simulink model "EvPowertrainController2EM"  (R2022b)
settings: configuration reference "VehicleFixed10ms" (kept outside this file)
model workspace (MAT data in the model file):
  CtrlVcuCnstrntPnltyFctr = 10000000
  CtrlVcuEMTrqSplitGrid = 200
  CtrlVcuPwrDeltaPnlty = 2
  CtrlVcuTracPwrErrPnlty = 6
  CtrlVcuTrqVecBrkThresh = 0.01
  CtrlVcuTrqVecIGain = 0
  CtrlVcuTrqVecMinTrq = 50
  CtrlVcuTrqVecPGain = -2000
  CtrlVcuTrqVecSteerThresh = 0.349065850399
  CtrlVcuTrqVecVelThresh = 2.5
undefined symbols (not defined in the file): AAM_IM_InvGrbx_Ploss, AAM_IM_spd, AAM_IM_TrqBrkPts, AAM_IPM_InvGrbx_Ploss, AAM_IPM_spd, AAM_IPM_TrqBrkPts, Bolt_n_map_spd, Bolt_n_map_trq, BrkPts_Spd, BrkPts_Trq, BrkPts_Vdc, CtrlVcuEvChrgLmtBpt, CtrlVcuEvRegenBrkCutOff, CtrlVcuEvRegenBrkSpdBpt, CtrlVcuEvSocBpt, eff, FrontDiffRatio, PlntBrkActrBoreFrnt, PlntBrkFrntBias, PlntBrkKinFricCffFrnt, PlntBrkNumPadsFrnt, PlntBrkPadMeanRadiusFrnt, PlntBrkPrsFctr, PlntBrkRearBias, PlntDiffrntl2Eff, PlntDiffrntl2Ratio, PlntDiffrntlEff, PlntDiffrntlRatio, PlntEM3Trq, PlntEMWhlGearEffFL, PlntEMWhlGearEffRL, PlntEMWhlGearRatioFL, PlntEMWhlGearRatioRL, PlntTransEffSpdBpt, PlntTransEffTbl, PlntTransEffTempBpt, PlntTransEffTrqBpt, PlntTransGearNumVect, PlntTransGearRatioVect, PlntWhlLdRadius, Ploss_AllVdc, RearDiffRatio, Spark_EffMap, Spark_MaxTrq, Spark_MaxTrq_Spd, Spark_Spd_BrkPts, Spark_Trq_BrkPts, SRM_DCVoltBrkPnt, SRM_InvGrbx_Ploss, SRM_op_TrqBrkPnt, SRM_Ploss_InvMotGrbx, SRM_SpdBrkPnt, SRM_TrqBrkPnt
libraries: simulink x7, autolibutils x2
(part 2 of 2)

== system EvPowertrainController2EM/Energy Management/Convert Whl to EMTrq Vector/2EM/Diff Eta1 ==
  note: Pwr >= 0, v = 1
      | Pwr < 0, v= -1
  SpdIn : Inport
  TrqIn : Inport  Port=2
  Constant : Constant  Value=PlntDiffrntl2Eff
  Constant1 : Constant  SampleTime=-1
  Constant2 : Constant  Value=-1  SampleTime=-1
  Math Function1 : Math  Operator=pow  SignedPower=on  OutputSignalType=real
  Product1 : Product
  Switch2 : Switch  SaturateOnIntegerOverflow=off  InputSameDT=off
  eta : Outport  VectorParamsAs1DForOutWhenUnconnected=off
  wires:
  TrqIn/1 -> Product1/1
  Math Function1/1 -> eta/1
  Switch2/1 -> Math Function1/2
  Product1/1 -> Switch2/2
  Constant1/1 -> Switch2/1
  Constant2/1 -> Switch2/3
  Constant/1 -> Math Function1/1
  SpdIn/1 -> Product1/2

== system EvPowertrainController2EM/Energy Management/Convert Whl to EMTrq Vector/3EM Dual Front/Diff Eta ==
  note: Pwr >= 0, v = 1
      | Pwr < 0, v= -1
  SpdIn : Inport
  TrqIn : Inport  Port=2
  Constant : Constant  Value=PlntDiffrntl2Eff
  Constant1 : Constant  SampleTime=-1
  Constant2 : Constant  Value=-1  SampleTime=-1
  Math Function1 : Math  Operator=pow  SignedPower=on  OutputSignalType=real
  Product1 : Product
  Switch2 : Switch  SaturateOnIntegerOverflow=off  InputSameDT=off
  eta : Outport  VectorParamsAs1DForOutWhenUnconnected=off
  wires:
  SpdIn/1 -> Product1/2
  Constant/1 -> Math Function1/1
  Constant2/1 -> Switch2/3
  Constant1/1 -> Switch2/1
  Product1/1 -> Switch2/2
  Switch2/1 -> Math Function1/2
  Math Function1/1 -> eta/1
  TrqIn/1 -> Product1/1

== system EvPowertrainController2EM/Energy Management/Convert Whl to EMTrq Vector/3EM Dual Front/Gear Eta ==
  note: Pwr >= 0, v = 1
      | Pwr < 0, v= -1
  SpdIn : Inport
  TrqIn : Inport  Port=2
  Constant : Constant  Value=PlntEMWhlGearEffFL
  Constant1 : Constant  SampleTime=-1
  Constant2 : Constant  Value=-1  SampleTime=-1
  Math Function1 : Math  Operator=pow  SignedPower=on  OutputSignalType=real
  Product1 : Product
  Switch2 : Switch  SaturateOnIntegerOverflow=off  InputSameDT=off
  eta : Outport  VectorParamsAs1DForOutWhenUnconnected=off
  wires:
  TrqIn/1 -> Product1/1
  Math Function1/1 -> eta/1
  Switch2/1 -> Math Function1/2
  Product1/1 -> Switch2/2
  Constant1/1 -> Switch2/1
  Constant2/1 -> Switch2/3
  Constant/1 -> Math Function1/1
  SpdIn/1 -> Product1/2

== system EvPowertrainController2EM/Energy Management/Convert Whl to EMTrq Vector/3EM Dual Rear/Diff Eta ==
  note: Pwr >= 0, v = 1
      | Pwr < 0, v= -1
  SpdIn : Inport
  TrqIn : Inport  Port=2
  Constant : Constant  Value=PlntDiffrntlEff
  Constant1 : Constant  SampleTime=-1
  Constant2 : Constant  Value=-1  SampleTime=-1
  Math Function1 : Math  Operator=pow  SignedPower=on  OutputSignalType=real
  Product1 : Product
  Switch2 : Switch  SaturateOnIntegerOverflow=off  InputSameDT=off
  eta : Outport  VectorParamsAs1DForOutWhenUnconnected=off
  wires:
  SpdIn/1 -> Product1/2
  Constant/1 -> Math Function1/1
  Constant2/1 -> Switch2/3
  Constant1/1 -> Switch2/1
  Product1/1 -> Switch2/2
  Switch2/1 -> Math Function1/2
  Math Function1/1 -> eta/1
  TrqIn/1 -> Product1/1

== system EvPowertrainController2EM/Energy Management/Convert Whl to EMTrq Vector/3EM Dual Rear/Gear Eta ==
  note: Pwr >= 0, v = 1
      | Pwr < 0, v= -1
  SpdIn : Inport
  TrqIn : Inport  Port=2
  Constant : Constant  Value=PlntEMWhlGearEffRL
  Constant1 : Constant  SampleTime=-1
  Constant2 : Constant  Value=-1  SampleTime=-1
  Math Function1 : Math  Operator=pow  SignedPower=on  OutputSignalType=real
  Product1 : Product
  Switch2 : Switch  SaturateOnIntegerOverflow=off  InputSameDT=off
  eta : Outport  VectorParamsAs1DForOutWhenUnconnected=off
  wires:
  TrqIn/1 -> Product1/1
  Math Function1/1 -> eta/1
  Switch2/1 -> Math Function1/2
  Product1/1 -> Switch2/2
  Constant1/1 -> Switch2/1
  Constant2/1 -> Switch2/3
  Constant/1 -> Math Function1/1
  SpdIn/1 -> Product1/2

== system EvPowertrainController2EM/Energy Management/Convert Whl to EMTrq Vector/4EM/Gear Eta ==
  note: Pwr >= 0, v = 1
      | Pwr < 0, v= -1
  SpdIn : Inport
  TrqIn : Inport  Port=2
  Constant : Constant  Value=PlntEMWhlGearEffFL
  Constant1 : Constant  SampleTime=-1
  Constant2 : Constant  Value=-1  SampleTime=-1
  Math Function1 : Math  Operator=pow  SignedPower=on  OutputSignalType=real
  Product1 : Product
  Switch2 : Switch  SaturateOnIntegerOverflow=off  InputSameDT=off
  eta : Outport  VectorParamsAs1DForOutWhenUnconnected=off
  wires:
  TrqIn/1 -> Product1/1
  Math Function1/1 -> eta/1
  Switch2/1 -> Math Function1/2
  Product1/1 -> Switch2/2
  Constant1/1 -> Switch2/1
  Constant2/1 -> Switch2/3
  Constant/1 -> Math Function1/1
  SpdIn/1 -> Product1/2

== system EvPowertrainController2EM/Energy Management/Convert Whl to EMTrq Vector/4EM/Gear Eta1 ==
  note: Pwr >= 0, v = 1
      | Pwr < 0, v= -1
  SpdIn : Inport
  TrqIn : Inport  Port=2
  Constant : Constant  Value=PlntEMWhlGearEffRL
  Constant1 : Constant  SampleTime=-1
  Constant2 : Constant  Value=-1  SampleTime=-1
  Math Function1 : Math  Operator=pow  SignedPower=on  OutputSignalType=real
  Product1 : Product
  Switch2 : Switch  SaturateOnIntegerOverflow=off  InputSameDT=off
  eta : Outport  VectorParamsAs1DForOutWhenUnconnected=off
  wires:
  SpdIn/1 -> Product1/2
  Constant/1 -> Math Function1/1
  Constant2/1 -> Switch2/3
  Constant1/1 -> Switch2/1
  Product1/1 -> Switch2/2
  Switch2/1 -> Math Function1/2
  Math Function1/1 -> eta/1
  TrqIn/1 -> Product1/1

== system EvPowertrainController2EM/Energy Management/Powertrain Constraints /Battery Constraint/Electrical Current ==
  BattV : Inport
  EMPwrElecVec : Inport  Port=2
  DC-DC Eta : Subsystem  Variant=on  VariantControlMode=label  VariantControl=Variant1  LabelModeActiveChoice=0
  Divide : Product  Inputs=*/
  Saturation : Saturate  UpperLimit=Inf  LowerLimit=0.0001
  BatteryAmp : Outport  VectorParamsAs1DForOutWhenUnconnected=off
  wires:
  DC-DC Eta/1(Out) -> Divide/1
  EMPwrElecVec/1 -> DC-DC Eta/1(In)
  Divide/1 -> BatteryAmp/1
  BattV/1 -> Saturation/1
  Saturation/1 -> Divide/2

== system EvPowertrainController2EM/Energy Management/Powertrain Constraints /Battery Constraint/Power Limit Calculations ==
  note: Use Current Limits from BMS to calculate
      | discharge and charge power limits
  BattPwrDisChrgLmt : Inport
  "BattPwrChrgLmt " : Inport  Port=2
  BattV_in : Inport  Port=3
  Data Type Conversion : DataTypeConversion  SaturateOnIntegerOverflow=off  RndMeth=Floor
  Data Type Conversion1 : DataTypeConversion  SaturateOnIntegerOverflow=off  RndMeth=Floor
  Divide : Product  Inputs=*/
  Divide1 : Product  Inputs=/*
  div0protect - poly : autolibutils/div0protect - poly  thresh=.01  ZeroCross=off  ZeroCross1=on  aMode=aMode
  div0protect - poly1 : autolibutils/div0protect - poly  thresh=.01  ZeroCross=off  ZeroCross1=on  aMode=aMode
  BattCurrDischrgLmt : Outport  VectorParamsAs1DForOutWhenUnconnected=off
  BattCurrChrgLmt : Outport  Port=2  VectorParamsAs1DForOutWhenUnconnected=off
  BattPwrDischrgLmt : Outport  Port=3  VectorParamsAs1DForOutWhenUnconnected=off
  BattPwrChrgLmt : Outport  Port=4  VectorParamsAs1DForOutWhenUnconnected=off
  wires:
  "BattPwrChrgLmt "/1 -> Divide1/2, Data Type Conversion/1
  BattPwrDisChrgLmt/1 -> Divide/1, Data Type Conversion1/1
  Data Type Conversion/1 -> BattPwrChrgLmt/1
  Data Type Conversion1/1 -> BattPwrDischrgLmt/1
  Divide/1 -> BattCurrDischrgLmt/1
  BattV_in/1 -> div0protect - poly/1, div0protect - poly1/1
  Divide1/1 -> BattCurrChrgLmt/1
  div0protect - poly/1 -> Divide1/1
  div0protect - poly1/1 -> Divide/2

== system EvPowertrainController2EM/Energy Management/Powertrain Constraints /EM Constraint Front/Maximum Torque ==
  note: Don't allow negative MotTrq when
      | WhlTrqCmd is >= 0
  WhlTrqCmd : Inport
  WhlEMTrqSplitVecFrnt : Inport  Port=2
  WhlTrqMaxVec : Inport  Port=3
  Compare To Zero : simulink/Logic and Bit Operations/Compare To Zero  relop=<  OutDataTypeStr=boolean
  Compare To Zero1 : simulink/Logic and Bit Operations/Compare To Zero  relop=>=  OutDataTypeStr=boolean
  Gain : Gain  Gain=-1
  Logical Operator : Logic  Operator=OR  Inputs=3  AllPortsSameDT=off  OutDataTypeStr=boolean
  Logical Operator1 : Logic  AllPortsSameDT=off  OutDataTypeStr=boolean
  Relational Operator : RelationalOperator  Operator=<  OutDataTypeStr=boolean  RndMeth=Simplest  InputSameDT=off
  Relational Operator1 : RelationalOperator  Operator=<  OutDataTypeStr=boolean  RndMeth=Simplest  InputSameDT=off
  Saturation Dynamic : simulink/Discontinuities/Saturation Dynamic  OutMin=[]  OutMax=[]  OutDataTypeStr=Inherit: Same as second input  OutDataType=fixdt(1, 16)  OutScaling=2^-10  DoSatur=off
  WhlEMTrqSatVec : Outport  VectorParamsAs1DForOutWhenUnconnected=off
  InfeasibleEMVec : Outport  Port=2  VectorParamsAs1DForOutWhenUnconnected=off
  wires:
  Logical Operator1/1 -> Logical Operator/3
  Compare To Zero1/1 -> Logical Operator1/2
  WhlEMTrqSplitVecFrnt/1 -> Relational Operator/2, Relational Operator1/1, Saturation Dynamic/2, Compare To Zero/1
  Compare To Zero/1 -> Logical Operator1/1
  WhlTrqCmd/1 -> Compare To Zero1/1
  Gain/1 -> Relational Operator1/2, Saturation Dynamic/3
  Saturation Dynamic/1 -> WhlEMTrqSatVec/1
  Relational Operator/1 -> Logical Operator/1
  Relational Operator1/1 -> Logical Operator/2
  Logical Operator/1 -> InfeasibleEMVec/1
  WhlTrqMaxVec/1 -> Gain/1, Relational Operator/1, Saturation Dynamic/1

== system EvPowertrainController2EM/Energy Management/Powertrain Constraints /EM Constraint Front/Tabular Power Loss Data ==
  EMAvgSpdVec : Inport
  WhlEMTrqSatVec : Inport  Port=2
  BatVin : Inport  Port=3
  2EM Stock : Subsystem  VariantControl=FrEff == 1
  2EM Team : Subsystem  VariantControl=FrEff == 2
  EMPwrElecVec : Outport

== system EvPowertrainController2EM/Energy Management/Powertrain Constraints /EM Constraint Rear/Maximum Torque ==
  note: Don't allow negative MotTrq when
      | WhlTrqCmd is >= 0
  WhlTrqCmd : Inport
  WhlEMTrqSplitVecRear : Inport  Port=2
  WhlTrqMaxVec : Inport  Port=3
  Compare To Zero : simulink/Logic and Bit Operations/Compare To Zero  relop=<  OutDataTypeStr=boolean
  Compare To Zero1 : simulink/Logic and Bit Operations/Compare To Zero  relop=>=  OutDataTypeStr=boolean
  Gain : Gain  Gain=-1
  Logical Operator : Logic  Operator=OR  Inputs=3  AllPortsSameDT=off  OutDataTypeStr=boolean
  Logical Operator1 : Logic  AllPortsSameDT=off  OutDataTypeStr=boolean
  Relational Operator : RelationalOperator  Operator=<  OutDataTypeStr=boolean  RndMeth=Simplest  InputSameDT=off
  Relational Operator1 : RelationalOperator  Operator=<  OutDataTypeStr=boolean  RndMeth=Simplest  InputSameDT=off
  Saturation Dynamic : simulink/Discontinuities/Saturation Dynamic  OutMin=[]  OutMax=[]  OutDataTypeStr=Inherit: Same as second input  OutDataType=fixdt(1, 16)  OutScaling=2^-10  DoSatur=off
  WhlEMTrqSatVec : Outport  VectorParamsAs1DForOutWhenUnconnected=off
  InfeasibleEMVec : Outport  Port=2  VectorParamsAs1DForOutWhenUnconnected=off
  wires:
  WhlTrqMaxVec/1 -> Saturation Dynamic/1, Relational Operator/1, Gain/1
  Logical Operator/1 -> InfeasibleEMVec/1
  Relational Operator1/1 -> Logical Operator/2
  Relational Operator/1 -> Logical Operator/1
  Saturation Dynamic/1 -> WhlEMTrqSatVec/1
  Gain/1 -> Saturation Dynamic/3, Relational Operator1/2
  WhlTrqCmd/1 -> Compare To Zero1/1
  Compare To Zero/1 -> Logical Operator1/1
  WhlEMTrqSplitVecRear/1 -> Compare To Zero/1, Saturation Dynamic/2, Relational Operator1/1, Relational Operator/2
  Compare To Zero1/1 -> Logical Operator1/2
  Logical Operator1/1 -> Logical Operator/3

== system EvPowertrainController2EM/Energy Management/Powertrain Constraints /EM Constraint Rear/Tabular Power Loss Data ==
  EMAvgSpdVec : Inport
  WhlEMTrqSatVec : Inport  Port=2
  BatVin : Inport  Port=3
  2EM Stock : Subsystem  VariantControl=RrEff == 1
  2EM Team : Subsystem  VariantControl=RrEff == 2
  EMPwrElecVec : Outport

== system EvPowertrainController2EM/Accel Pedal to Traction Wheel Torque Request/2EM/EMTrq2WhlTrqFrnt/No Transmission/Diff Eta ==
  note: Pwr >= 0, v = 1
      | Pwr < 0, v= -1
  SpdIn : Inport
  TrqIn : Inport  Port=2
  Constant : Constant  Value=PlntDiffrntlEff
  Constant1 : Constant  SampleTime=-1
  Constant2 : Constant  Value=-1  SampleTime=-1
  Math Function1 : Math  Operator=pow  SignedPower=on  OutputSignalType=real
  Product1 : Product
  Switch2 : Switch  SaturateOnIntegerOverflow=off  InputSameDT=off
  eta : Outport  VectorParamsAs1DForOutWhenUnconnected=off
  wires:
  SpdIn/1 -> Product1/2
  Constant/1 -> Math Function1/1
  Constant2/1 -> Switch2/3
  Constant1/1 -> Switch2/1
  Product1/1 -> Switch2/2
  Switch2/1 -> Math Function1/2
  Math Function1/1 -> eta/1
  TrqIn/1 -> Product1/1

== system EvPowertrainController2EM/Accel Pedal to Traction Wheel Torque Request/2EM/EMTrq2WhlTrqFrnt/Transmission/Diff Eta ==
  SpdIn : Inport
  TrqIn : Inport  Port=2
  Constant : Constant  Value=PlntDiffrntlEff
  Constant1 : Constant  SampleTime=-1
  Constant2 : Constant  Value=-1  SampleTime=-1
  Math Function1 : Math  Operator=pow  SignedPower=on  OutputSignalType=real
  Product1 : Product
  Switch2 : Switch  SaturateOnIntegerOverflow=off  InputSameDT=off
  eta : Outport  VectorParamsAs1DForOutWhenUnconnected=off
  wires:
  SpdIn/1 -> Product1/2
  Constant/1 -> Math Function1/1
  Constant2/1 -> Switch2/3
  Constant1/1 -> Switch2/1
  Product1/1 -> Switch2/2
  Switch2/1 -> Math Function1/2
  Math Function1/1 -> eta/1
  TrqIn/1 -> Product1/1

== system EvPowertrainController2EM/Accel Pedal to Traction Wheel Torque Request/2EM/EMTrq2WhlTrqFrnt/Transmission/Trans Eta ==
  TrqIn : Inport
  SpdIn : Inport  Port=2
  Gear : Inport  Port=3
  Abs1 : Abs  SaturateOnIntegerOverflow=off
  Constant : Constant  Value=PlntTransEffTempBpt(1)
  Constant1 : Constant  SampleTime=-1
  Constant2 : Constant  Value=-1  SampleTime=-1
  Eta 4D : Lookup_n-D  NumberOfTableDimensions=4  LookupTableObject=''  BreakpointsForDimension1=PlntTransEffTrqBpt  BreakpointsForDimension2=PlntTransEffSpdBpt  BreakpointsForDimension3=PlntTransGearNumVect  BreakpointsForDimension4=PlntTransEffTempBpt  Table=PlntTransEffTbl  ExtrapMethod=Clip  InternalRulePriority=Speed  RndMeth=Simplest
      settings: InputPortMap=u0,u1,u2,u3
  Math Function1 : Math  Operator=pow  SignedPower=on  OutputSignalType=real
  Product1 : Product
  Switch2 : Switch  SaturateOnIntegerOverflow=off  InputSameDT=off
  eta : Outport  VectorParamsAs1DForOutWhenUnconnected=off
  wires:
  TrqIn/1 -> Product1/1, Abs1/1
  Math Function1/1 -> eta/1
  Abs1/1 -> Eta 4D/1
  Switch2/1 -> Math Function1/2
  Product1/1 -> Switch2/2
  Constant1/1 -> Switch2/1
  Constant2/1 -> Switch2/3
  Eta 4D/1 -> Math Function1/1
  SpdIn/1 -> Product1/2, Eta 4D/2
  Gear/1 -> Eta 4D/3
  Constant/1 -> Eta 4D/4

== system EvPowertrainController2EM/Accel Pedal to Traction Wheel Torque Request/2EM/EMTrq2WhlTrqRear/No Transmission/Diff Eta ==
  note: Pwr >= 0, v = 1
      | Pwr < 0, v= -1
  SpdIn : Inport
  TrqIn : Inport  Port=2
  Constant : Constant  Value=PlntDiffrntl2Eff
  Constant1 : Constant  SampleTime=-1
  Constant2 : Constant  Value=-1  SampleTime=-1
  Math Function1 : Math  Operator=pow  SignedPower=on  OutputSignalType=real
  Product1 : Product
  Switch2 : Switch  SaturateOnIntegerOverflow=off  InputSameDT=off
  eta : Outport  VectorParamsAs1DForOutWhenUnconnected=off
  wires:
  SpdIn/1 -> Product1/2
  Constant/1 -> Math Function1/1
  Constant2/1 -> Switch2/3
  Constant1/1 -> Switch2/1
  Product1/1 -> Switch2/2
  Switch2/1 -> Math Function1/2
  Math Function1/1 -> eta/1
  TrqIn/1 -> Product1/1

== system EvPowertrainController2EM/Accel Pedal to Traction Wheel Torque Request/2EM/EMTrq2WhlTrqRear/Transmission/Diff Eta ==
  SpdIn : Inport
  TrqIn : Inport  Port=2
  Constant : Constant  Value=PlntDiffrntl2Eff
  Constant1 : Constant  SampleTime=-1
  Constant2 : Constant  Value=-1  SampleTime=-1
  Math Function1 : Math  Operator=pow  SignedPower=on  OutputSignalType=real
  Product1 : Product
  Switch2 : Switch  SaturateOnIntegerOverflow=off  InputSameDT=off
  eta : Outport  VectorParamsAs1DForOutWhenUnconnected=off
  wires:
  TrqIn/1 -> Product1/1
  Math Function1/1 -> eta/1
  Switch2/1 -> Math Function1/2
  Product1/1 -> Switch2/2
  Constant1/1 -> Switch2/1
  Constant2/1 -> Switch2/3
  Constant/1 -> Math Function1/1
  SpdIn/1 -> Product1/2

== system EvPowertrainController2EM/Accel Pedal to Traction Wheel Torque Request/2EM/EMTrq2WhlTrqRear/Transmission/Trans Eta ==
  TrqIn : Inport
  SpdIn : Inport  Port=2
  Gear : Inport  Port=3
  Abs1 : Abs  SaturateOnIntegerOverflow=off
  Constant : Constant  Value=PlntTransEffTempBpt(1)
  Constant1 : Constant  SampleTime=-1
  Constant2 : Constant  Value=-1  SampleTime=-1
  Eta 4D : Lookup_n-D  NumberOfTableDimensions=4  LookupTableObject=''  BreakpointsForDimension1=PlntTransEffTrqBpt  BreakpointsForDimension2=PlntTransEffSpdBpt  BreakpointsForDimension3=PlntTransGearNumVect  BreakpointsForDimension4=PlntTransEffTempBpt  Table=PlntTransEffTbl  ExtrapMethod=Clip  InternalRulePriority=Speed  RndMeth=Simplest
      settings: InputPortMap=u0,u1,u2,u3
  Math Function1 : Math  Operator=pow  SignedPower=on  OutputSignalType=real
  Product1 : Product
  Switch2 : Switch  SaturateOnIntegerOverflow=off  InputSameDT=off
  eta : Outport  VectorParamsAs1DForOutWhenUnconnected=off
  wires:
  Constant/1 -> Eta 4D/4
  Gear/1 -> Eta 4D/3
  SpdIn/1 -> Eta 4D/2, Product1/2
  Eta 4D/1 -> Math Function1/1
  Constant2/1 -> Switch2/3
  Constant1/1 -> Switch2/1
  Product1/1 -> Switch2/2
  Switch2/1 -> Math Function1/2
  Abs1/1 -> Eta 4D/1
  Math Function1/1 -> eta/1
  TrqIn/1 -> Abs1/1, Product1/1

== system EvPowertrainController2EM/Energy Management/2EM/EMTrq2WhlTrqFrnt/No Transmission/Diff Eta ==
  note: Pwr >= 0, v = 1
      | Pwr < 0, v= -1
  SpdIn : Inport
  TrqIn : Inport  Port=2
  Constant : Constant  Value=PlntDiffrntlEff
  Constant1 : Constant  SampleTime=-1
  Constant2 : Constant  Value=-1  SampleTime=-1
  Math Function1 : Math  Operator=pow  SignedPower=on  OutputSignalType=real
  Product1 : Product
  Switch2 : Switch  SaturateOnIntegerOverflow=off  InputSameDT=off
  eta : Outport  VectorParamsAs1DForOutWhenUnconnected=off
  wires:
  SpdIn/1 -> Product1/2
  Constant/1 -> Math Function1/1
  Constant2/1 -> Switch2/3
  Constant1/1 -> Switch2/1
  Product1/1 -> Switch2/2
  Switch2/1 -> Math Function1/2
  Math Function1/1 -> eta/1
  TrqIn/1 -> Product1/1

== system EvPowertrainController2EM/Energy Management/2EM/EMTrq2WhlTrqFrnt/Transmission/Diff Eta ==
  SpdIn : Inport
  TrqIn : Inport  Port=2
  Constant : Constant  Value=PlntDiffrntlEff
  Constant1 : Constant  SampleTime=-1
  Constant2 : Constant  Value=-1  SampleTime=-1
  Math Function1 : Math  Operator=pow  SignedPower=on  OutputSignalType=real
  Product1 : Product
  Switch2 : Switch  SaturateOnIntegerOverflow=off  InputSameDT=off
  eta : Outport  VectorParamsAs1DForOutWhenUnconnected=off
  wires:
  SpdIn/1 -> Product1/2
  Constant/1 -> Math Function1/1
  Constant2/1 -> Switch2/3
  Constant1/1 -> Switch2/1
  Product1/1 -> Switch2/2
  Switch2/1 -> Math Function1/2
  Math Function1/1 -> eta/1
  TrqIn/1 -> Product1/1

== system EvPowertrainController2EM/Energy Management/2EM/EMTrq2WhlTrqFrnt/Transmission/Trans Eta ==
  TrqIn : Inport
  SpdIn : Inport  Port=2
  Gear : Inport  Port=3
  Abs1 : Abs  SaturateOnIntegerOverflow=off
  Constant : Constant  Value=PlntTransEffTempBpt(1)
  Constant1 : Constant  SampleTime=-1
  Constant2 : Constant  Value=-1  SampleTime=-1
  Eta 4D : Lookup_n-D  NumberOfTableDimensions=4  LookupTableObject=''  BreakpointsForDimension1=PlntTransEffTrqBpt  BreakpointsForDimension2=PlntTransEffSpdBpt  BreakpointsForDimension3=PlntTransGearNumVect  BreakpointsForDimension4=PlntTransEffTempBpt  Table=PlntTransEffTbl  ExtrapMethod=Clip  InternalRulePriority=Speed  RndMeth=Simplest
      settings: InputPortMap=u0,u1,u2,u3
  Math Function1 : Math  Operator=pow  SignedPower=on  OutputSignalType=real
  Product1 : Product
  Switch2 : Switch  SaturateOnIntegerOverflow=off  InputSameDT=off
  eta : Outport  VectorParamsAs1DForOutWhenUnconnected=off
  wires:
  TrqIn/1 -> Product1/1, Abs1/1
  Math Function1/1 -> eta/1
  Abs1/1 -> Eta 4D/1
  Switch2/1 -> Math Function1/2
  Product1/1 -> Switch2/2
  Constant1/1 -> Switch2/1
  Constant2/1 -> Switch2/3
  Eta 4D/1 -> Math Function1/1
  SpdIn/1 -> Product1/2, Eta 4D/2
  Gear/1 -> Eta 4D/3
  Constant/1 -> Eta 4D/4

== system EvPowertrainController2EM/Energy Management/2EM/EMTrq2WhlTrqRear/No Transmission/Diff Eta ==
  note: Pwr >= 0, v = 1
      | Pwr < 0, v= -1
  SpdIn : Inport
  TrqIn : Inport  Port=2
  Constant : Constant  Value=PlntDiffrntl2Eff
  Constant1 : Constant  SampleTime=-1
  Constant2 : Constant  Value=-1  SampleTime=-1
  Math Function1 : Math  Operator=pow  SignedPower=on  OutputSignalType=real
  Product1 : Product
  Switch2 : Switch  SaturateOnIntegerOverflow=off  InputSameDT=off
  eta : Outport  VectorParamsAs1DForOutWhenUnconnected=off
  wires:
  SpdIn/1 -> Product1/2
  Constant/1 -> Math Function1/1
  Constant2/1 -> Switch2/3
  Constant1/1 -> Switch2/1
  Product1/1 -> Switch2/2
  Switch2/1 -> Math Function1/2
  Math Function1/1 -> eta/1
  TrqIn/1 -> Product1/1

== system EvPowertrainController2EM/Energy Management/2EM/EMTrq2WhlTrqRear/Transmission/Diff Eta ==
  SpdIn : Inport
  TrqIn : Inport  Port=2
  Constant : Constant  Value=PlntDiffrntl2Eff
  Constant1 : Constant  SampleTime=-1
  Constant2 : Constant  Value=-1  SampleTime=-1
  Math Function1 : Math  Operator=pow  SignedPower=on  OutputSignalType=real
  Product1 : Product
  Switch2 : Switch  SaturateOnIntegerOverflow=off  InputSameDT=off
  eta : Outport  VectorParamsAs1DForOutWhenUnconnected=off
  wires:
  TrqIn/1 -> Product1/1
  Math Function1/1 -> eta/1
  Switch2/1 -> Math Function1/2
  Product1/1 -> Switch2/2
  Constant1/1 -> Switch2/1
  Constant2/1 -> Switch2/3
  Constant/1 -> Math Function1/1
  SpdIn/1 -> Product1/2

== system EvPowertrainController2EM/Energy Management/2EM/EMTrq2WhlTrqRear/Transmission/Trans Eta ==
  TrqIn : Inport
  SpdIn : Inport  Port=2
  Gear : Inport  Port=3
  Abs1 : Abs  SaturateOnIntegerOverflow=off
  Constant : Constant  Value=PlntTransEffTempBpt(1)
  Constant1 : Constant  SampleTime=-1
  Constant2 : Constant  Value=-1  SampleTime=-1
  Eta 4D : Lookup_n-D  NumberOfTableDimensions=4  LookupTableObject=''  BreakpointsForDimension1=PlntTransEffTrqBpt  BreakpointsForDimension2=PlntTransEffSpdBpt  BreakpointsForDimension3=PlntTransGearNumVect  BreakpointsForDimension4=PlntTransEffTempBpt  Table=PlntTransEffTbl  ExtrapMethod=Clip  InternalRulePriority=Speed  RndMeth=Simplest
      settings: InputPortMap=u0,u1,u2,u3
  Math Function1 : Math  Operator=pow  SignedPower=on  OutputSignalType=real
  Product1 : Product
  Switch2 : Switch  SaturateOnIntegerOverflow=off  InputSameDT=off
  eta : Outport  VectorParamsAs1DForOutWhenUnconnected=off
  wires:
  Constant/1 -> Eta 4D/4
  Gear/1 -> Eta 4D/3
  SpdIn/1 -> Eta 4D/2, Product1/2
  Eta 4D/1 -> Math Function1/1
  Constant2/1 -> Switch2/3
  Constant1/1 -> Switch2/1
  Product1/1 -> Switch2/2
  Switch2/1 -> Math Function1/2
  Abs1/1 -> Eta 4D/1
  Math Function1/1 -> eta/1
  TrqIn/1 -> Abs1/1, Product1/1

== system EvPowertrainController2EM/Energy Management/Control Domain /Rear Axle EM Torque Vector/2EM or 3EM Dual Front/Diff Eta ==
  note: Pwr >= 0, v = 1
      | Pwr < 0, v= -1
  SpdIn : Inport
  TrqIn : Inport  Port=2
  Constant : Constant  Value=PlntDiffrntl2Eff
  Constant1 : Constant  SampleTime=-1
  Constant2 : Constant  Value=-1  SampleTime=-1
  Math Function1 : Math  Operator=pow  SignedPower=on  OutputSignalType=real
  Product1 : Product
  Switch2 : Switch  SaturateOnIntegerOverflow=off  InputSameDT=off
  eta : Outport  VectorParamsAs1DForOutWhenUnconnected=off
  wires:
  SpdIn/1 -> Product1/2
  Constant/1 -> Math Function1/1
  Constant2/1 -> Switch2/3
  Constant1/1 -> Switch2/1
  Product1/1 -> Switch2/2
  Switch2/1 -> Math Function1/2
  Math Function1/1 -> eta/1
  TrqIn/1 -> Product1/1

== system EvPowertrainController2EM/Energy Management/Control Domain /Rear Axle EM Torque Vector/3EM Dual Rear or 4EM/Gear Eta ==
  note: Pwr >= 0, v = 1
      | Pwr < 0, v= -1
  SpdIn : Inport
  TrqIn : Inport  Port=2
  Constant : Constant  Value=PlntEMWhlGearEffRL
  Constant1 : Constant  SampleTime=-1
  Constant2 : Constant  Value=-1  SampleTime=-1
  Math Function1 : Math  Operator=pow  SignedPower=on  OutputSignalType=real
  Product1 : Product
  Switch2 : Switch  SaturateOnIntegerOverflow=off  InputSameDT=off
  eta : Outport  VectorParamsAs1DForOutWhenUnconnected=off
  wires:
  SpdIn/1 -> Product1/2
  Constant/1 -> Math Function1/1
  Constant2/1 -> Switch2/3
  Constant1/1 -> Switch2/1
  Product1/1 -> Switch2/2
  Switch2/1 -> Math Function1/2
  Math Function1/1 -> eta/1
  TrqIn/1 -> Product1/1

== system EvPowertrainController2EM/Energy Management/Powertrain Constraints /Battery Constraint/Electrical Current/DC-DC Eta ==
  In : Inport
  DC-DC Eta : Subsystem  VariantControl=1
  No DC-DC : Subsystem  VariantControl=0
  Out : Outport  VectorParamsAs1DForOutWhenUnconnected=off

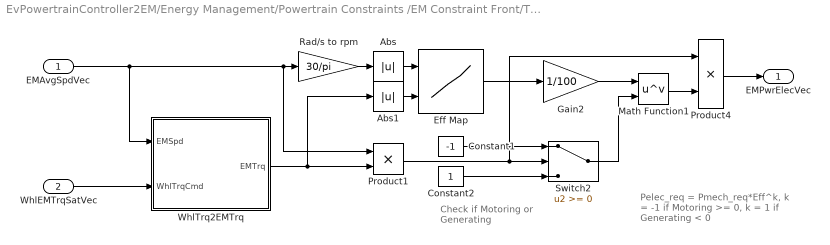
== system EvPowertrainController2EM/Energy Management/Powertrain Constraints /EM Constraint Front/Tabular Power Loss Data/2EM Stock ==
  note: Pelec_req = Pmech_req*Eff^k,
      | k = -1 if Motoring >= 0,
      | k = 1 if Generating < 0
  note: Check if Motoring
      | or Generating
  EMAvgSpdVec : Inport
  WhlEMTrqSatVec : Inport  Port=2
  Abs : Abs  SaturateOnIntegerOverflow=off
  Abs1 : Abs  SaturateOnIntegerOverflow=off
  Constant1 : Constant  Value=-1  SampleTime=-1
  Constant2 : Constant  SampleTime=-1
  Eff Map : Lookup_n-D  BreakpointsForDimension1=Spark_Spd_BrkPts  BreakpointsForDimension2=Spark_Trq_BrkPts  IndexSearchMethod=Linear search  BeginIndexSearchUsingPreviousIndexResult=on  Table=Spark_EffMap  UseLastTableValue=on  InternalRulePriority=Speed  OutDataTypeStr=Inherit: Inherit from 'Table data'  RndMeth=Simplest
      settings: InputPortMap=u0,u1
  Gain2 : Gain  Gain=1/100
  Math Function1 : Math  Operator=pow  SignedPower=on  OutputSignalType=real
  Product1 : Product
  Product4 : Product
  Rad/s to rpm : Gain  Gain=30/pi
  Switch2 : Switch  SaturateOnIntegerOverflow=off  InputSameDT=off
  WhlTrq2EMTrq : Subsystem  VariantControl=2EM or 3EMDualFront
  EMPwrElecVec : Outport  VectorParamsAs1DForOutWhenUnconnected=off
  wires:
  WhlEMTrqSatVec/1 -> WhlTrq2EMTrq/2(WhlTrqCmd)
  EMAvgSpdVec/1 -> Product1/1, Rad/s to rpm/1, WhlTrq2EMTrq/1(EMSpd)
  Eff Map/1 -> Gain2/1
  Abs1/1 -> Eff Map/2
  Abs/1 -> Eff Map/1
  Gain2/1 -> Math Function1/1
  Constant2/1 -> Switch2/3
  Constant1/1 -> Switch2/1
  Product1/1 -> Switch2/2, Product4/1
  Switch2/1 -> Math Function1/2
  Math Function1/1 -> Product4/2
  Product4/1 -> EMPwrElecVec/1
  WhlTrq2EMTrq/1(EMTrq) -> Abs1/1, Product1/2
  Rad/s to rpm/1 -> Abs/1

== system EvPowertrainController2EM/Energy Management/Powertrain Constraints /EM Constraint Front/Tabular Power Loss Data/2EM Team ==
  note: Check if Motoring
      | or Generating
  note: Pelec_req = Pmech_req*Eff^k,
      | k = -1 if Motoring >= 0,
      | k = 1 if Generating < 0
  EMAvgSpdVec : Inport
  WhlEMTrqSatVec : Inport  Port=2
  BatVin : Inport  Port=3
  Abs : Abs  SaturateOnIntegerOverflow=off
  Abs1 : Abs  SaturateOnIntegerOverflow=off
  Constant1 : Constant  Value=-1  SampleTime=-1
  Constant2 : Constant  SampleTime=-1
  Product : Product
  Product1 : Product
  Subsystem : Subsystem  Variant=on  VariantControl=Choice
      settings: PortSchema="{\"entries\":[{\"content\":{\"sides\":[{\"content\":{\"connectorIds\":[\"In1\",\"In2\"]},\"type\":\"ConnectorPlacement.EquallySpacedRectSide\",\"uuid\":\"c6a41dad-f1d6-44fe-a3bd-a7fb60924ac2\"},{\"content\":{\"connectorIds\":[\"Out1\"],\"side\":\"RIGHT\"},\"type\":\"ConnectorPlacement.EquallySpacedRectSide\",\"uuid\":\"4aa94d7b-905a-48f8-8a33-a07e39c9bb79\"},{\"content\":{\"connectorIds\":[],\"side\":\"TOP\"},\"type\":\"ConnectorPlacement.EquallySpacedRectSide\",\"uuid\":\"f9efebd2-8088-45fc-b274-a0855bc368e5\"},{\"content\":{\"connectorIds\":[\"In3\"],\"side\":\"BOTTOM\"},\"type\":\"ConnectorPlacement.EquallySpacedRectSide\",\"uuid\":\"2a3bcf5d-0492-4b31-9d5b-8c1953178a15\"}]},\"type\":\"ConnectorPlacement.EquallySpacedConnector\",\"uuid\":\"6c009010-9d89-4498-a9bb-72f2068edef5\"}],\"packageUris\":[\"http://schema.mathworks.com/mf0/Connector/R2020b\"],\"version\":\"1.0\"}"
  Subtract : Sum  Inputs=+-
  Switch2 : Switch  SaturateOnIntegerOverflow=off  InputSameDT=off
  WhlTrq2EMTrq : Subsystem  VariantControl=2EM or 3EMDualFront
  EMPwrElecVec : Outport  VectorParamsAs1DForOutWhenUnconnected=off
  wires:
  WhlTrq2EMTrq/1(EMTrq) -> Product1/2, Abs1/1
  Subtract/1 -> EMPwrElecVec/1
  Switch2/1 -> Product/2
  Product1/1 -> Subtract/1, Switch2/2
  Constant1/1 -> Switch2/1
  Constant2/1 -> Switch2/3
  Product/1 -> Subtract/2
  Abs/1 -> Subsystem/1(In1)
  Abs1/1 -> Subsystem/2(In2)
  Subsystem/1(Out1) -> Product/1
  EMAvgSpdVec/1 -> Abs/1, Product1/1, WhlTrq2EMTrq/1(EMSpd)
  WhlEMTrqSatVec/1 -> WhlTrq2EMTrq/2(WhlTrqCmd)
  BatVin/1 -> Subsystem/3(BatVin)

== system EvPowertrainController2EM/Energy Management/Powertrain Constraints /EM Constraint Rear/Tabular Power Loss Data/2EM Stock ==
  note: Pelec_req = Pmech_req*Eff^k,
      | k = -1 if Motoring >= 0,
      | k = 1 if Generating < 0
  note: Check if Motoring
      | or Generating
  EMAvgSpdVec : Inport
  WhlEMTrqSatVec : Inport  Port=2
  Abs : Abs  SaturateOnIntegerOverflow=off
  Abs1 : Abs  SaturateOnIntegerOverflow=off
  Constant1 : Constant  Value=-1  SampleTime=-1
  Constant2 : Constant  SampleTime=-1
  Eff Map : Lookup_n-D  BreakpointsForDimension1=Spark_Spd_BrkPts  BreakpointsForDimension2=Spark_Trq_BrkPts  IndexSearchMethod=Linear search  BeginIndexSearchUsingPreviousIndexResult=on  Table=Spark_EffMap  UseLastTableValue=on  InternalRulePriority=Speed  OutDataTypeStr=Inherit: Inherit from 'Table data'  RndMeth=Simplest
      settings: InputPortMap=u0,u1
  Gain2 : Gain  Gain=1/100
  Math Function1 : Math  Operator=pow  SignedPower=on  OutputSignalType=real
  Product1 : Product
  Product4 : Product
  Rad/s to rpm : Gain  Gain=30/pi
  Switch2 : Switch  SaturateOnIntegerOverflow=off  InputSameDT=off
  WhlTrq2EMTrq : Subsystem  VariantControl=2EM or 3EMDualFront
  EMPwrElecVec : Outport  VectorParamsAs1DForOutWhenUnconnected=off
  wires:
  WhlEMTrqSatVec/1 -> WhlTrq2EMTrq/2(WhlTrqCmd)
  EMAvgSpdVec/1 -> WhlTrq2EMTrq/1(EMSpd), Product1/1, Rad/s to rpm/1
  Eff Map/1 -> Gain2/1  "Rear Eff"
  Abs1/1 -> Eff Map/2
  Abs/1 -> Eff Map/1
  Gain2/1 -> Math Function1/1
  Constant2/1 -> Switch2/3
  Constant1/1 -> Switch2/1
  Product1/1 -> Switch2/2, Product4/1
  Switch2/1 -> Math Function1/2
  Math Function1/1 -> Product4/2
  Product4/1 -> EMPwrElecVec/1
  WhlTrq2EMTrq/1(EMTrq) -> Abs1/1, Product1/2
  Rad/s to rpm/1 -> Abs/1

== system EvPowertrainController2EM/Energy Management/Powertrain Constraints /EM Constraint Rear/Tabular Power Loss Data/2EM Team ==
  note: Check if Motoring
      | or Generating
  note: Pelec_req = Pmech_req*Eff^k,
      | k = -1 if Motoring >= 0,
      | k = 1 if Generating < 0
  EMAvgSpdVec : Inport
  WhlEMTrqSatVec : Inport  Port=2
  BatVin : Inport  Port=3
  Abs : Abs  SaturateOnIntegerOverflow=off
  Abs1 : Abs  SaturateOnIntegerOverflow=off
  Constant1 : Constant  Value=-1  SampleTime=-1
  Constant2 : Constant  SampleTime=-1
  Product : Product
  Product1 : Product
  Subsystem : Subsystem  Variant=on  VariantControl=Choice
      settings: PortSchema="{\"entries\":[{\"content\":{\"sides\":[{\"content\":{\"connectorIds\":[\"In1\",\"In2\"]},\"type\":\"ConnectorPlacement.EquallySpacedRectSide\",\"uuid\":\"c6a41dad-f1d6-44fe-a3bd-a7fb60924ac2\"},{\"content\":{\"connectorIds\":[\"Out1\"],\"side\":\"RIGHT\"},\"type\":\"ConnectorPlacement.EquallySpacedRectSide\",\"uuid\":\"4aa94d7b-905a-48f8-8a33-a07e39c9bb79\"},{\"content\":{\"connectorIds\":[],\"side\":\"TOP\"},\"type\":\"ConnectorPlacement.EquallySpacedRectSide\",\"uuid\":\"f9efebd2-8088-45fc-b274-a0855bc368e5\"},{\"content\":{\"connectorIds\":[\"In3\"],\"side\":\"BOTTOM\"},\"type\":\"ConnectorPlacement.EquallySpacedRectSide\",\"uuid\":\"2a3bcf5d-0492-4b31-9d5b-8c1953178a15\"}]},\"type\":\"ConnectorPlacement.EquallySpacedConnector\",\"uuid\":\"6c009010-9d89-4498-a9bb-72f2068edef5\"}],\"packageUris\":[\"http://schema.mathworks.com/mf0/Connector/R2020b\"],\"version\":\"1.0\"}"
  Subtract : Sum  Inputs=+-
  Switch2 : Switch  SaturateOnIntegerOverflow=off  InputSameDT=off
  WhlTrq2EMTrq : Subsystem  VariantControl=2EM or 3EMDualFront
  EMPwrElecVec : Outport  VectorParamsAs1DForOutWhenUnconnected=off
  wires:
  WhlTrq2EMTrq/1(EMTrq) -> Abs1/1, Product1/2
  Subtract/1 -> EMPwrElecVec/1
  Switch2/1 -> Product/2
  Product1/1 -> Subtract/1, Switch2/2
  Constant1/1 -> Switch2/1
  Constant2/1 -> Switch2/3
  EMAvgSpdVec/1 -> Abs/1, Product1/1, WhlTrq2EMTrq/1(EMSpd)
  WhlEMTrqSatVec/1 -> WhlTrq2EMTrq/2(WhlTrqCmd)
  Product/1 -> Subtract/2
  BatVin/1 -> Subsystem/3(BatVin)
  Abs/1 -> Subsystem/1(In1)
  Abs1/1 -> Subsystem/2(In2)
  Subsystem/1(Out1) -> Product/1

== system EvPowertrainController2EM/Energy Management/Powertrain Constraints /Battery Constraint/Electrical Current/DC-DC Eta/DC-DC Eta ==
  In : Inport
  DCDC Constant Eff : Gain  Gain=1+(100-eff)/100
  Out : Outport  VectorParamsAs1DForOutWhenUnconnected=off
  wires:
  DCDC Constant Eff/1 -> Out/1
  In/1 -> DCDC Constant Eff/1

== system EvPowertrainController2EM/Energy Management/Powertrain Constraints /Battery Constraint/Electrical Current/DC-DC Eta/No DC-DC ==
  In : Inport
  Out : Outport  VectorParamsAs1DForOutWhenUnconnected=off
  wires:
  In/1 -> Out/1

== system EvPowertrainController2EM/Energy Management/Powertrain Constraints /EM Constraint Front/Tabular Power Loss Data/2EM Stock/WhlTrq2EMTrq ==
  EMSpd : Inport
  WhlTrqCmd : Inport  Port=2
  Diff Eta : Subsystem
  Divide2 : Product  Inputs=/*
  Gain3 : Gain  Gain=1/PlntDiffrntlRatio
  Unit Delay : UnitDelay  SampleTime=-1  HasFrameUpgradeWarning=on
  EMTrq : Outport  VectorParamsAs1DForOutWhenUnconnected=off
  wires:
  Unit Delay/1 -> Diff Eta/2(TrqIn)
  Diff Eta/1(eta) -> Divide2/1
  WhlTrqCmd/1 -> Gain3/1
  EMSpd/1 -> Diff Eta/1(SpdIn)
  Divide2/1 -> EMTrq/1, Unit Delay/1
  Gain3/1 -> Divide2/2

== system EvPowertrainController2EM/Energy Management/Powertrain Constraints /EM Constraint Front/Tabular Power Loss Data/2EM Team/Subsystem ==
  In1 : Inport
  In2 : Inport  Port=2
  BatVin : Inport  Port=3
  AAM IM : Subsystem  VariantControl=em1 == 3
  AAM IPM : Subsystem  VariantControl=em1 == 2
  Trillium SRM : Subsystem  VariantControl=em1 == 4
  Trillium SRM(+) : Subsystem  VariantControl=em1 == 6
  YASA P400HC : Subsystem  VariantControl=em1 == 5
  Out1 : Outport

== system EvPowertrainController2EM/Energy Management/Powertrain Constraints /EM Constraint Front/Tabular Power Loss Data/2EM Team/WhlTrq2EMTrq ==
  EMSpd : Inport
  WhlTrqCmd : Inport  Port=2
  Diff Eta : Subsystem
  Divide2 : Product  Inputs=/*
  Gain3 : Gain  Gain=1/FrontDiffRatio
  Unit Delay : UnitDelay  SampleTime=-1  HasFrameUpgradeWarning=on
  EMTrq : Outport  VectorParamsAs1DForOutWhenUnconnected=off
  wires:
  Gain3/1 -> Divide2/2
  Divide2/1 -> Unit Delay/1, EMTrq/1
  EMSpd/1 -> Diff Eta/1(SpdIn)
  WhlTrqCmd/1 -> Gain3/1
  Diff Eta/1(eta) -> Divide2/1
  Unit Delay/1 -> Diff Eta/2(TrqIn)

== system EvPowertrainController2EM/Energy Management/Powertrain Constraints /EM Constraint Rear/Tabular Power Loss Data/2EM Stock/WhlTrq2EMTrq ==
  EMSpd : Inport
  WhlTrqCmd : Inport  Port=2
  Diff Eta : Subsystem
  Divide2 : Product  Inputs=/*
  Gain3 : Gain  Gain=1/PlntDiffrntl2Ratio
  Unit Delay : UnitDelay  SampleTime=-1  HasFrameUpgradeWarning=on
  EMTrq : Outport  VectorParamsAs1DForOutWhenUnconnected=off
  wires:
  Unit Delay/1 -> Diff Eta/2(TrqIn)
  Diff Eta/1(eta) -> Divide2/1
  WhlTrqCmd/1 -> Gain3/1
  EMSpd/1 -> Diff Eta/1(SpdIn)
  Divide2/1 -> EMTrq/1, Unit Delay/1
  Gain3/1 -> Divide2/2

== system EvPowertrainController2EM/Energy Management/Powertrain Constraints /EM Constraint Rear/Tabular Power Loss Data/2EM Team/Subsystem ==
  In1 : Inport
  In2 : Inport  Port=2
  BatVin : Inport  Port=3
  AAM IM : Subsystem  VariantControl=em2 == 3
  AAM IPM : Subsystem  VariantControl=em2 == 2
  Bolt IPM : Subsystem  VariantControl=em2 == 6
  Trillium SRM : Subsystem  VariantControl=em2 == 5
  Trillium SRM(+) : Subsystem  VariantControl=em2 == 4
  Out1 : Outport

== system EvPowertrainController2EM/Energy Management/Powertrain Constraints /EM Constraint Rear/Tabular Power Loss Data/2EM Team/WhlTrq2EMTrq ==
  EMSpd : Inport
  WhlTrqCmd : Inport  Port=2
  Diff Eta : Subsystem
  Divide2 : Product  Inputs=/*
  Gain2 : Gain  Gain=1/RearDiffRatio
  Unit Delay : UnitDelay  SampleTime=-1  HasFrameUpgradeWarning=on
  EMTrq : Outport  VectorParamsAs1DForOutWhenUnconnected=off
  wires:
  Gain2/1 -> Divide2/2
  Divide2/1 -> Unit Delay/1, EMTrq/1
  EMSpd/1 -> Diff Eta/1(SpdIn)
  WhlTrqCmd/1 -> Gain2/1
  Diff Eta/1(eta) -> Divide2/1
  Unit Delay/1 -> Diff Eta/2(TrqIn)

== system EvPowertrainController2EM/Energy Management/Powertrain Constraints /EM Constraint Front/Tabular Power Loss Data/2EM Stock/WhlTrq2EMTrq/Diff Eta ==
  note: Pwr >= 0, v = 1
      | Pwr < 0, v= -1
  SpdIn : Inport
  TrqIn : Inport  Port=2
  Constant : Constant  Value=PlntDiffrntl2Eff
  Constant1 : Constant  SampleTime=-1
  Constant2 : Constant  Value=-1  SampleTime=-1
  Math Function1 : Math  Operator=pow  SignedPower=on  OutputSignalType=real
  Product1 : Product
  Switch2 : Switch  SaturateOnIntegerOverflow=off  InputSameDT=off
  eta : Outport  VectorParamsAs1DForOutWhenUnconnected=off
  wires:
  SpdIn/1 -> Product1/2
  Constant/1 -> Math Function1/1
  Constant2/1 -> Switch2/3
  Constant1/1 -> Switch2/1
  Product1/1 -> Switch2/2
  Switch2/1 -> Math Function1/2
  Math Function1/1 -> eta/1
  TrqIn/1 -> Product1/1

== system EvPowertrainController2EM/Energy Management/Powertrain Constraints /EM Constraint Front/Tabular Power Loss Data/2EM Team/Subsystem/AAM IM ==
  In1 : Inport
  In2 : Inport  Port=2
  Loss Map : Lookup_n-D  BreakpointsForDimension1=AAM_IM_spd  BreakpointsForDimension2=AAM_IM_TrqBrkPts  BeginIndexSearchUsingPreviousIndexResult=on  Table=AAM_IM_InvGrbx_Ploss  ExtrapMethod=Clip  UseLastTableValue=on  InternalRulePriority=Speed  OutDataTypeStr=Inherit: Inherit from 'Table data'  RndMeth=Simplest
      settings: InputPortMap=u0,u1
  Out1 : Outport
  wires:
  In1/1 -> Loss Map/1
  Loss Map/1 -> Out1/1
  In2/1 -> Loss Map/2

== system EvPowertrainController2EM/Energy Management/Powertrain Constraints /EM Constraint Front/Tabular Power Loss Data/2EM Team/Subsystem/AAM IPM ==
  In1 : Inport
  In2 : Inport  Port=2
  Loss Map : Lookup_n-D  BreakpointsForDimension1=AAM_IPM_spd  BreakpointsForDimension2=AAM_IPM_TrqBrkPts  BeginIndexSearchUsingPreviousIndexResult=on  Table=AAM_IPM_InvGrbx_Ploss  ExtrapMethod=Clip  UseLastTableValue=on  InternalRulePriority=Speed  OutDataTypeStr=Inherit: Inherit from 'Table data'  RndMeth=Simplest
      settings: InputPortMap=u0,u1
  Out1 : Outport
  wires:
  In2/1 -> Loss Map/2
  Loss Map/1 -> Out1/1
  In1/1 -> Loss Map/1

== system EvPowertrainController2EM/Energy Management/Powertrain Constraints /EM Constraint Front/Tabular Power Loss Data/2EM Team/Subsystem/Trillium SRM ==
  In1 : Inport
  In2 : Inport  Port=2
  BatVin : Inport  Port=3
  Loss Map : Lookup_n-D  NumberOfTableDimensions=3  BreakpointsForDimension1=SRM_SpdBrkPnt  BreakpointsForDimension2=SRM_TrqBrkPnt  BreakpointsForDimension3=SRM_DCVoltBrkPnt  BeginIndexSearchUsingPreviousIndexResult=on  Table=SRM_InvGrbx_Ploss  ExtrapMethod=Clip  UseLastTableValue=on  InternalRulePriority=Speed  OutDataTypeStr=Inherit: Inherit from 'Table data'  RndMeth=Simplest
      settings: InputPortMap=u0,u1,u2
  Out1 : Outport
  wires:
  In2/1 -> Loss Map/2
  Loss Map/1 -> Out1/1
  In1/1 -> Loss Map/1
  BatVin/1 -> Loss Map/3

== system EvPowertrainController2EM/Energy Management/Powertrain Constraints /EM Constraint Front/Tabular Power Loss Data/2EM Team/Subsystem/Trillium SRM(+) ==
  In1 : Inport
  In2 : Inport  Port=2
  BatVin : Inport  Port=3
  Loss Map : Lookup_n-D  BreakpointsForDimension1=SRM_op_TrqBrkPnt  BreakpointsForDimension2=SRM_SpdBrkPnt  BreakpointsForDimension3=SRM_DCVoltBrkPnt  BeginIndexSearchUsingPreviousIndexResult=on  Table=SRM_Ploss_InvMotGrbx  ExtrapMethod=Clip  UseLastTableValue=on  InternalRulePriority=Speed  OutDataTypeStr=Inherit: Inherit from 'Table data'  RndMeth=Simplest
      settings: InputPortMap=u0,u1
  Terminator : Terminator
  Out1 : Outport
  wires:
  In2/1 -> Loss Map/2
  Loss Map/1 -> Out1/1
  In1/1 -> Loss Map/1
  BatVin/1 -> Terminator/1

== system EvPowertrainController2EM/Energy Management/Powertrain Constraints /EM Constraint Front/Tabular Power Loss Data/2EM Team/Subsystem/YASA P400HC ==
  In1 : Inport
  In2 : Inport  Port=2
  BatVin : Inport  Port=3
  Loss Map : Lookup_n-D  NumberOfTableDimensions=3  BreakpointsForDimension1=BrkPts_Trq  BreakpointsForDimension2=BrkPts_Spd  BreakpointsForDimension3=BrkPts_Vdc  BeginIndexSearchUsingPreviousIndexResult=on  Table=Ploss_AllVdc  ExtrapMethod=Clip  UseLastTableValue=on  InternalRulePriority=Speed  OutDataTypeStr=Inherit: Inherit from 'Table data'  RndMeth=Simplest
      settings: InputPortMap=u0,u1,u2
  Out1 : Outport
  wires:
  BatVin/1 -> Loss Map/3
  In1/1 -> Loss Map/1
  Loss Map/1 -> Out1/1
  In2/1 -> Loss Map/2

== system EvPowertrainController2EM/Energy Management/Powertrain Constraints /EM Constraint Front/Tabular Power Loss Data/2EM Team/WhlTrq2EMTrq/Diff Eta ==
  note: Pwr >= 0, v = 1
      | Pwr < 0, v= -1
  SpdIn : Inport
  TrqIn : Inport  Port=2
  Constant : Constant  Value=PlntDiffrntl2Eff
  Constant1 : Constant  SampleTime=-1
  Constant2 : Constant  Value=-1  SampleTime=-1
  Math Function1 : Math  Operator=pow  SignedPower=on  OutputSignalType=real
  Product1 : Product
  Switch2 : Switch  SaturateOnIntegerOverflow=off  InputSameDT=off
  eta : Outport  VectorParamsAs1DForOutWhenUnconnected=off
  wires:
  TrqIn/1 -> Product1/1
  Math Function1/1 -> eta/1
  Switch2/1 -> Math Function1/2
  Product1/1 -> Switch2/2
  Constant1/1 -> Switch2/1
  Constant2/1 -> Switch2/3
  Constant/1 -> Math Function1/1
  SpdIn/1 -> Product1/2

== system EvPowertrainController2EM/Energy Management/Powertrain Constraints /EM Constraint Rear/Tabular Power Loss Data/2EM Stock/WhlTrq2EMTrq/Diff Eta ==
  note: Pwr >= 0, v = 1
      | Pwr < 0, v= -1
  SpdIn : Inport
  TrqIn : Inport  Port=2
  Constant : Constant  Value=PlntDiffrntl2Eff
  Constant1 : Constant  SampleTime=-1
  Constant2 : Constant  Value=-1  SampleTime=-1
  Math Function1 : Math  Operator=pow  SignedPower=on  OutputSignalType=real
  Product1 : Product
  Switch2 : Switch  SaturateOnIntegerOverflow=off  InputSameDT=off
  eta : Outport  VectorParamsAs1DForOutWhenUnconnected=off
  wires:
  SpdIn/1 -> Product1/2
  Constant/1 -> Math Function1/1
  Constant2/1 -> Switch2/3
  Constant1/1 -> Switch2/1
  Product1/1 -> Switch2/2
  Switch2/1 -> Math Function1/2
  Math Function1/1 -> eta/1
  TrqIn/1 -> Product1/1

== system EvPowertrainController2EM/Energy Management/Powertrain Constraints /EM Constraint Rear/Tabular Power Loss Data/2EM Team/Subsystem/AAM IM ==
  In1 : Inport
  In2 : Inport  Port=2
  Loss Map : Lookup_n-D  BreakpointsForDimension1=AAM_IM_spd  BreakpointsForDimension2=AAM_IM_TrqBrkPts  BeginIndexSearchUsingPreviousIndexResult=on  Table=AAM_IM_InvGrbx_Ploss  ExtrapMethod=Clip  UseLastTableValue=on  InternalRulePriority=Speed  OutDataTypeStr=Inherit: Inherit from 'Table data'  RndMeth=Simplest
      settings: InputPortMap=u0,u1
  Out1 : Outport
  wires:
  In1/1 -> Loss Map/1
  Loss Map/1 -> Out1/1
  In2/1 -> Loss Map/2

== system EvPowertrainController2EM/Energy Management/Powertrain Constraints /EM Constraint Rear/Tabular Power Loss Data/2EM Team/Subsystem/AAM IPM ==
  In1 : Inport
  In2 : Inport  Port=2
  Loss Map : Lookup_n-D  BreakpointsForDimension1=AAM_IPM_spd  BreakpointsForDimension2=AAM_IPM_TrqBrkPts  BeginIndexSearchUsingPreviousIndexResult=on  Table=AAM_IPM_InvGrbx_Ploss  ExtrapMethod=Clip  UseLastTableValue=on  InternalRulePriority=Speed  OutDataTypeStr=Inherit: Inherit from 'Table data'  RndMeth=Simplest
      settings: InputPortMap=u0,u1
  Out1 : Outport
  wires:
  In2/1 -> Loss Map/2
  Loss Map/1 -> Out1/1
  In1/1 -> Loss Map/1

== system EvPowertrainController2EM/Energy Management/Powertrain Constraints /EM Constraint Rear/Tabular Power Loss Data/2EM Team/Subsystem/Bolt IPM ==
  In1 : Inport
  In2 : Inport  Port=2
  Loss Map : Lookup_n-D  BreakpointsForDimension1=Bolt_n_map_trq  BreakpointsForDimension2=Bolt_n_map_spd  BreakpointsForDimension3=BrkPts_Vdc  BeginIndexSearchUsingPreviousIndexResult=on  Table=Bolt_LossMap/0.975/0.98  ExtrapMethod=Clip  UseLastTableValue=on  InternalRulePriority=Speed  OutDataTypeStr=Inherit: Inherit from 'Table data'  RndMeth=Simplest
      settings: InputPortMap=u0,u1
  Out1 : Outport
  wires:
  In2/1 -> Loss Map/1
  Loss Map/1 -> Out1/1
  In1/1 -> Loss Map/2

== system EvPowertrainController2EM/Energy Management/Powertrain Constraints /EM Constraint Rear/Tabular Power Loss Data/2EM Team/Subsystem/Trillium SRM ==
  In1 : Inport
  In2 : Inport  Port=2
  BatVin : Inport  Port=3
  Loss Map : Lookup_n-D  NumberOfTableDimensions=3  BreakpointsForDimension1=SRM_SpdBrkPnt  BreakpointsForDimension2=SRM_TrqBrkPnt  BreakpointsForDimension3=SRM_DCVoltBrkPnt  BeginIndexSearchUsingPreviousIndexResult=on  Table=SRM_InvGrbx_Ploss  ExtrapMethod=Clip  UseLastTableValue=on  InternalRulePriority=Speed  OutDataTypeStr=Inherit: Inherit from 'Table data'  RndMeth=Simplest
      settings: InputPortMap=u0,u1,u2
  Out1 : Outport
  wires:
  In1/1 -> Loss Map/1
  Loss Map/1 -> Out1/1
  In2/1 -> Loss Map/2
  BatVin/1 -> Loss Map/3

== system EvPowertrainController2EM/Energy Management/Powertrain Constraints /EM Constraint Rear/Tabular Power Loss Data/2EM Team/Subsystem/Trillium SRM(+) ==
  In1 : Inport
  In2 : Inport  Port=2
  BatVin : Inport  Port=3
  Loss Map : Lookup_n-D  BreakpointsForDimension1=SRM_op_TrqBrkPnt  BreakpointsForDimension2=SRM_SpdBrkPnt  BreakpointsForDimension3=SRM_DCVoltBrkPnt  BeginIndexSearchUsingPreviousIndexResult=on  Table=SRM_Ploss_InvMotGrbx  ExtrapMethod=Clip  UseLastTableValue=on  InternalRulePriority=Speed  OutDataTypeStr=Inherit: Inherit from 'Table data'  RndMeth=Simplest
      settings: InputPortMap=u0,u1
  Terminator : Terminator
  Out1 : Outport
  wires:
  In2/1 -> Loss Map/2
  Loss Map/1 -> Out1/1
  In1/1 -> Loss Map/1
  BatVin/1 -> Terminator/1

== system EvPowertrainController2EM/Energy Management/Powertrain Constraints /EM Constraint Rear/Tabular Power Loss Data/2EM Team/WhlTrq2EMTrq/Diff Eta ==
  note: Pwr >= 0, v = 1
      | Pwr < 0, v= -1
  SpdIn : Inport
  TrqIn : Inport  Port=2
  Constant : Constant  Value=PlntDiffrntl2Eff
  Constant1 : Constant  SampleTime=-1
  Constant2 : Constant  Value=-1  SampleTime=-1
  Math Function1 : Math  Operator=pow  SignedPower=on  OutputSignalType=real
  Product1 : Product
  Switch2 : Switch  SaturateOnIntegerOverflow=off  InputSameDT=off
  eta : Outport  VectorParamsAs1DForOutWhenUnconnected=off
  wires:
  TrqIn/1 -> Product1/1
  Math Function1/1 -> eta/1
  Switch2/1 -> Math Function1/2
  Product1/1 -> Switch2/2
  Constant1/1 -> Switch2/1
  Constant2/1 -> Switch2/3
  Constant/1 -> Math Function1/1
  SpdIn/1 -> Product1/2

== matlab function EvPowertrainController2EM/Energy Management/Hamiltonian computation and minimization/MATLAB Function ==
  data: minH output; idx output; H input; InfFlag input; allInf output
function [minH, idx, allInf] = fcn(H, InfFlag)

if all(InfFlag) 
    [minH, idx] = min(H);
    allInf = 1;
else
    [minH, idx] = min(H);
    allInf = 0;
end
